simulink model "HW6_Simulink"  (R2019b)
settings: Solver=FixedStepAuto  StartTime=0.0  StopTime=20  RelTol=1e-3
InitFcn:
  | load('BusDefinitions.mat')
undefined symbols (not defined in the file): A1, A1_eval, A2_cont, A2_eval, B1, B1_eval, B2_cont, B2_eval, C1, C1_eval, C2_cont, C2_eval, codertarget, D1, D1_eval, D2_cont, D2_eval, DiscIntNeverNeededParam, Discrete, L1, L2, L3, L4, L5, q1_noise, q2_noise, q3_noise, q4_noise, q5_noise, r1_noise, r2_noise, r3_noise, r4_noise, r5_noise, Time, Ts
libraries: ctrlSharedLib x5, simulink x1
settings Model: ExtModeTrigDuration=80  Creator=Sankalp Bhan  LastModifiedBy=cwhipp
settings DataIOCC: SaveFormat=Structure
settings OptimizationCC: PassReuseOutputArgsThreshold=0  MaxStackSize=64
settings DebuggingCC: ParameterTunabilityLossMsg=error  ArithmeticOperatorsInVariantConditions=warning
settings HardwareCC: ProdBitPerPointer=32  ProdBitPerSizeT=32  ProdBitPerPtrDiffT=32  ProdLargestAtomicInteger=Long  ProdWordSize=32  ProdHWDeviceType=ARM Compatible->ARM 9  UseEmbeddedCoderFeatures=off
settings SFSimCC: SimUseLocalCustomCode=off  MATLABDynamicMemAlloc=off
settings RTWCC: SystemTargetFile=ert.tlc  HardwareBoard=PARROT Mambo  TLCOptions="-aInlineSetEventsForThisBaseRateFcn=TLC_FALSE -aSuppressMultiTaskScheduler=TLC_FALSE   -aRateBasedStepFcn=1"  TemplateMakefile=ert_default_tmf  GenerateReport=on  RTWUseLocalCustomCode=off  Toolchain=Sourcery G++ Lite GNU Toolchain for Drones  LaunchReport=on
settings CodeAppCC: ForceParamTrailComments=on  OperatorAnnotations=on  StateflowObjectComments=on
settings ERTTargetCC: ERTCustomFileBanners=off  MatFileLogging=on  SupportContinuousTime=on  SupportNonInlinedSFcns=on  RemoveResetFunc=off  ModelStepFunctionPrototypeControlCompliant=off

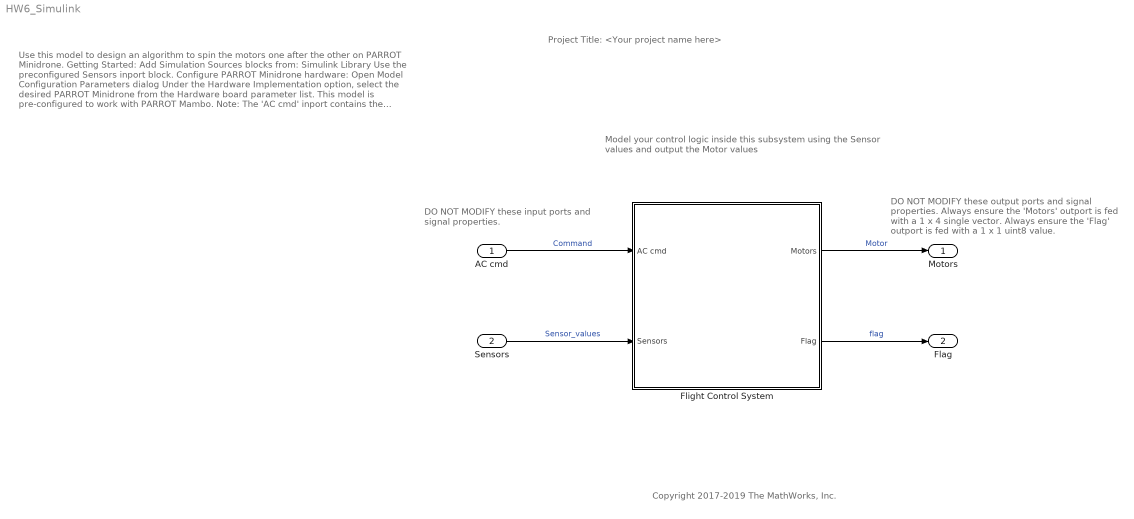
== system HW6_Simulink ==
  note: Model your control logic inside this subsystem
      | using the Sensor values and output the
      | Motor values
  note: DO NOT MODIFY these output ports
      | and signal properties.
      |
      |
      |
      | Always ensure the 'Motors' outport
      | is fed with a 1 x 4 single vector.
      |
      |
      |
      |
      |
      | Always ensure the 'Flag' outport is
      | fed with a 1 x 1 uint8 value.
  note: DO NOT MODIFY these input
      | ports and signal properties.
  note: Copyright 2017-2019 The MathWorks, Inc.
  note: Use this model to design an algorithm to spin the motors one
      | after the other on PARROT Minidrone.
      |
      | Getting Started:
      |
      | Add Simulation Sources blocks from:
      | Simulink Library
      | Use the preconfigured Sensors inport block.
      |
      | Configure PARROT Minidrone hardware:
      |
      | Open Model Configuration Parameters dialog
      |
      | Under the Hardware Implementation option, select the desired
      | PARROT Minidrone from the Hardware board parameter list.
      |
      | This model is pre-configured to work with PARROT Mambo.
      |
      | Note:
      |
      | The 'AC cmd' inport contains the position and orientation
      | reference signals information.
      | The 'Sensors' inport contains data from accelerometer,
      | gyroscope, ultrasonic, pressure and optical flow data.
      | The 'Flag' outport can be used to model an error condition
      | which stops the drone.
      | The 'Motors' outport is fed with the speed values of the 4 motors.
      | Learn more:
      |
      | Simulink Subsystem
      | Simulink Buses
  note: Project Title: <Your project name here>
  AC cmd : Inport  OutDataTypeStr=Bus: CommandBus  BusOutputAsStruct=on
  Sensors : Inport  Port=2  OutDataTypeStr=Bus: SensorsBus  BusOutputAsStruct=on
  Flight Control System : Subsystem  InitFcn=codertarget.parrot.internal.fcsSubsystemCallback(gcb);
  Motors : Outport  OutDataTypeStr=single  PortDimensions=[1 4]  VectorParamsAs1DForOutWhenUnconnected=off
  Flag : Outport  Port=2  OutDataTypeStr=uint8  PortDimensions=1  VectorParamsAs1DForOutWhenUnconnected=off
  wires:
  Flight Control System/1(Motors) -> Motors/1  "Motor"
  AC cmd/1 -> Flight Control System/1(AC cmd)  "Command"
  Sensors/1 -> Flight Control System/2(Sensors)  "Sensor_values"
  Flight Control System/2(Flag) -> Flag/1  "flag"

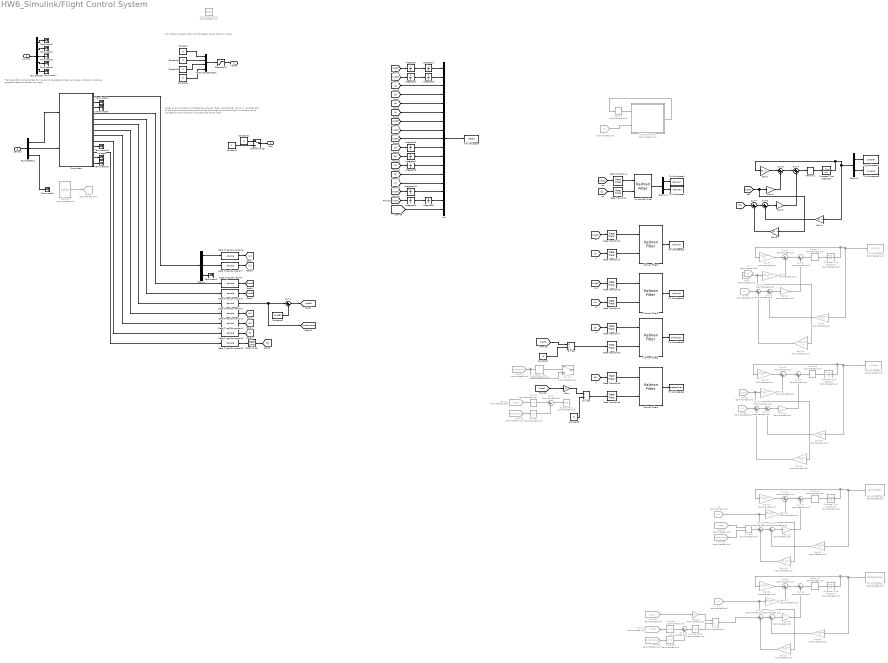
== system HW6_Simulink/Flight Control System ==
  note: The 'Motors' outport is fed with the speed values of the 4 motors.
  note: Model an error condition and feed the value to 'Flag' outport block.
      | Value '0' indicates that all the flight conditions are good and the drone
      | can continue its flight.
      | A non-zero value indicates an error condition, and stops the drone
      | flight.
  note: The SensorsBus contains data from sensors like
      | accelerometer, gyroscope, ultrasonic, pressure,
      | magnetometer and optical flow data.
  AC cmd : Inport
  Sensors : Inport  Port=2
  Bus Selector : BusSelector  OutputSignals=controlModePosVSOrient,pos_ref,takeoff_flag,orient_ref,live_time_ticks
  Bus Selector1 : BusSelector  OutputSignals=VisionSensors,HALSensors,SensorCalibration
  Constant{,3..5} (4 alike) : Constant  Value=0  SampleTime=0.005
  Constant1 : Constant  OutDataTypeStr=uint8
  Constant2 : Constant  Value=0  OutDataTypeStr=uint8
  Constant6 : Constant  Value=-9.4351
  Constant7 : Constant  Value=3
  Constant8 : Constant  Value=3
  Data Type Conversion{,1..8} (9 alike) : DataTypeConversion  OutDataTypeStr=double
  Demux : Demux  Outputs=3
  Demux1 : Demux  Outputs=2
  Demux2 : Demux  Outputs=2
  Discrete-Time Integrator : DiscreteIntegrator  IntegratorMethod=Integration: Backward Euler  SampleTime=-1  ICPrevOutput=DiscIntNeverNeededParam  ICPrevScaledInput=DiscIntNeverNeededParam
  Discrete-Time Integrator{1..4} (4 alike) : DiscreteIntegrator  Commented=on  IntegratorMethod=Integration: Backward Euler  SampleTime=-1  ICPrevOutput=DiscIntNeverNeededParam  ICPrevScaledInput=DiscIntNeverNeededParam
  Divide : Product  Inputs=*/
  Divide1 : Product  Inputs=*/
  Divide2 : Product  Commented=on  Inputs=*/
  Divide4 : Product  Commented=on  Inputs=*/
  From17 : From  Commented=on  GotoTag=vdot
  From{20,22..23,28} (4 alike) : From  Commented=on  GotoTag=wdotnobias
  From21 : From  Commented=on  GotoTag=vdot
  From26 : From  Commented=on  GotoTag=udot
  From27 : From  Commented=on  GotoTag=vdot
  Gain : Gain  Gain=-1
  Gain1 : Gain  Gain=A1  Multiplication=Matrix(K*u)
  Gain{10..11,16,21} (4 alike) : Gain  Commented=on  Gain=D2_cont  Multiplication=Matrix(K*u)
  Gain{5,12,17,22} (4 alike) : Gain  Commented=on  Gain=A2_cont  Multiplication=Matrix(K*u)
  Gain{7,13,18,23} (4 alike) : Gain  Commented=on  Gain=B2_cont  Multiplication=Matrix(K*u)
  Gain14 : Gain  Commented=on  Gain=L3  Multiplication=Matrix(K*u)
  Gain{9,15,20,25} (4 alike) : Gain  Commented=on  Gain=C2_cont  Multiplication=Matrix(K*u)
  Gain19 : Gain  Commented=on  Gain=L4  Multiplication=Matrix(K*u)
  Gain2 : Gain  Gain=B1  Multiplication=Matrix(K*u)
  Gain24 : Gain  Commented=on  Gain=L5  Multiplication=Matrix(K*u)
  Gain26 : Gain  Commented=on  Gain=-1
  Gain3 : Gain  Gain=L1  Multiplication=Matrix(K*u)
  Gain4 : Gain  Gain=C1  Multiplication=Matrix(K*u)
  Gain6 : Gain  Gain=D1  Multiplication=Matrix(K*u)
  Gain8 : Gain  Commented=on  Gain=L2  Multiplication=Matrix(K*u)
  Goto9 : Goto  Commented=on  GotoTag=azbias
  Integrator{,1..8,11} (10 alike) : Integrator
  Interval Test : simulink/Logic and Bit Operations/Interval Test  Commented=on  IntervalClosedRight=on  uplimit=0.5  IntervalClosedLeft=on  lowlimit=-0.5  OutDataTypeStr=boolean
  Kalman Filter1 : ctrlSharedLib/Kalman Filter  TimeDomain=Discrete-Time  UseCurrentEstimator=on  ModelSource=Individual A, B, C, D matrices  ModelSourceVariable=ss(0.95,1,1,0,1)  A=A2_eval  B=B2_eval  C=C2_eval  D=D2_eval  NumberOfStates=1  NumberOfInputs=1  NumberOfOutputs=1  InitialEstimateSource=Dialog  X0=[0]  P0=10  UseK=off  UseGH=off  NumberOfProcessNoiseInputs=1  G=1  TimeInvariantG=on  H=0  TimeInvariantH=on  Q=q2_noise;  TimeInvariantQ=on  R=r2_noise;  TimeInvariantR=on  N=0  TimeInvariantN=on  AddInputPort=on  AddEnablePort=off  OutputEstimatedY=off  OutputP=off  Ts=-1
      settings: SourceProductBaseCode=CT
  Kalman Filter2 : ctrlSharedLib/Kalman Filter  TimeDomain=Discrete-Time  UseCurrentEstimator=on  ModelSource=Individual A, B, C, D matrices  ModelSourceVariable=ss(0.95,1,1,0,1)  A=A2_eval  B=B2_eval  C=C2_eval  D=D2_eval  NumberOfStates=1  NumberOfInputs=1  NumberOfOutputs=1  InitialEstimateSource=Dialog  X0=[0]  P0=10  UseK=off  UseGH=off  NumberOfProcessNoiseInputs=1  G=1  TimeInvariantG=on  H=0  TimeInvariantH=on  Q=q3_noise;  TimeInvariantQ=on  R=r3_noise;  TimeInvariantR=on  N=0  TimeInvariantN=on  AddInputPort=on  AddEnablePort=off  OutputEstimatedY=off  OutputP=off  Ts=-1
      settings: SourceProductBaseCode=CT
  Kalman Filter3 : ctrlSharedLib/Kalman Filter  TimeDomain=Discrete-Time  UseCurrentEstimator=on  ModelSource=Individual A, B, C, D matrices  ModelSourceVariable=ss(0.95,1,1,0,1)  A=A2_eval  B=B2_eval  C=C2_eval  D=D2_eval  NumberOfStates=1  NumberOfInputs=1  NumberOfOutputs=1  InitialEstimateSource=Dialog  X0=[0]  P0=10  UseK=off  UseGH=off  NumberOfProcessNoiseInputs=1  G=1  TimeInvariantG=on  H=0  TimeInvariantH=on  Q=q4_noise;  TimeInvariantQ=on  R=r4_noise;  TimeInvariantR=on  N=0  TimeInvariantN=on  AddInputPort=on  AddEnablePort=off  OutputEstimatedY=off  OutputP=off  Ts=-1
      settings: SourceProductBaseCode=CT
  Kalman Filter4 : ctrlSharedLib/Kalman Filter  TimeDomain=Discrete-Time  UseCurrentEstimator=on  ModelSource=Individual A, B, C, D matrices  ModelSourceVariable=ss(0.95,1,1,0,1)  A=A2_eval  B=B2_eval  C=C2_eval  D=D2_eval  NumberOfStates=1  NumberOfInputs=1  NumberOfOutputs=1  InitialEstimateSource=Dialog  X0=[0]  P0=10  UseK=off  UseGH=off  NumberOfProcessNoiseInputs=1  G=1  TimeInvariantG=on  H=0  TimeInvariantH=on  Q=q5_noise;  TimeInvariantQ=on  R=r5_noise;  TimeInvariantR=on  N=0  TimeInvariantN=on  AddInputPort=on  AddEnablePort=off  OutputEstimatedY=off  OutputP=off  Ts=-1
      settings: SourceProductBaseCode=CT
  MATLAB Function : MATLAB Function  Commented=on  TreatAsAtomicUnit=on
  Manual Switch : ManualSwitch
  Memory{,2..5} (5 alike) : Memory  Commented=on
  Memory1 : Memory
  Mux : Mux  Inputs=17
  Pulse Generator2 : DiscretePulseGenerator  Commented=on  Amplitude=400  Period=1600  PulseWidth=400  PhaseDelay=1200  SampleTime=Ts
  Rate Limiter : RateLimiter  RisingSlewLimit=50  FallingSlewLimit=-50  SampleTimeMode=inherited
  Rate Transition{,1..9} (10 alike) : RateTransition  OutPortSampleTime=0.005
  Saturation1 : Saturate  UpperLimit=500  LowerLimit=0  OutDataTypeStr=single
  Selector : Selector  Commented=on  InputPortWidth=8  IndexOptions=Index vector (dialog)  Indices=[3]  OutputSizes=1
  Square{,1..3} (4 alike) : Math  Commented=on  Operator=square  SignedPower=off  SaturateOnIntegerOverflow=on
  Square Root : Sqrt  Commented=on  SaturateOnIntegerOverflow=on
  Square Root1 : Sqrt  Commented=on  SaturateOnIntegerOverflow=on
  Subsystem : Subsystem
  Sum1 : Sum  Inputs=|+-
  Sum{9..11,14..15,18..19,22} (8 alike) : Sum  Commented=on  Inputs=|+-
  Sum{2,6,8,12..13,16..17,20..21,23} (10 alike) : Sum  Commented=on  Inputs=|++
  Sum3 : Sum  Inputs=|++
  Sum4 : Sum  Inputs=|++
  Sum5 : Sum  Inputs=|+-
  Sum7 : Sum  Inputs=|+-
  Switch : Switch  Commented=on  Criteria=u2 > Threshold
  Terminator{1..9,15,18} (11 alike) : Terminator
  To Workspace : ToWorkspace  VariableName=states  SaveFormat=Structure With Time  SampleTime=-1
  To Workspace1 : ToWorkspace  VariableName=zkalman  SaveFormat=Structure With Time  SampleTime=-1
  To Workspace10 : ToWorkspace  Commented=on  VariableName=vwiener  SaveFormat=Structure With Time  SampleTime=-1
  To Workspace11 : ToWorkspace  Commented=on  VariableName=phiwiener  SaveFormat=Structure With Time  SampleTime=-1
  To Workspace12 : ToWorkspace  Commented=on  VariableName=thetawiener  SaveFormat=Structure With Time  SampleTime=-1
  To Workspace2 : ToWorkspace  VariableName=wkalman  SaveFormat=Structure With Time  SampleTime=-1
  To Workspace3 : ToWorkspace  VariableName=ukalman  SaveFormat=Structure With Time  SampleTime=-1
  To Workspace4 : ToWorkspace  VariableName=vkalman  SaveFormat=Structure With Time  SampleTime=-1
  To Workspace5 : ToWorkspace  VariableName=phikalman  SaveFormat=Structure With Time  SampleTime=-1
  To Workspace6 : ToWorkspace  VariableName=thetakalman  SaveFormat=Structure With Time  SampleTime=-1
  To Workspace7 : ToWorkspace  VariableName=zwiener  SaveFormat=Structure With Time  SampleTime=-1
  To Workspace8 : ToWorkspace  VariableName=wwiener  SaveFormat=Structure With Time  SampleTime=-1
  To Workspace9 : ToWorkspace  Commented=on  VariableName=uwiener  SaveFormat=Structure With Time  SampleTime=-1
  Vector Concatenate1 : Concatenate  NumInputs=4
  hello : From  Commented=on  GotoTag=udot
  hello1 : From  Commented=on  GotoTag=vdot
  its me : From  Commented=on  GotoTag=u
  its me1 : From  Commented=on  GotoTag=v
  p1 : From  Commented=on  GotoTag=p
  p2 : From  Commented=on  GotoTag=p
  q1 : From  Commented=on  GotoTag=q
  voltage : Terminator
  z : From  Commented=on  GotoTag=h
  zw Kalman Filter : ctrlSharedLib/Kalman Filter  TimeDomain=Discrete-Time  UseCurrentEstimator=on  ModelSource=Individual A, B, C, D matrices  ModelSourceVariable=ss(0.95,1,1,0,1)  A=A1_eval  B=B1_eval  C=C1_eval  D=D1_eval  NumberOfStates=1  NumberOfInputs=1  NumberOfOutputs=1  InitialEstimateSource=Dialog  X0=[0;0 ]  P0=10  UseK=off  UseGH=off  NumberOfProcessNoiseInputs=1  G=1  TimeInvariantG=on  H=0  TimeInvariantH=on  Q=[0 0 ; 0 1].*q1_noise;  TimeInvariantQ=on  R=r1_noise;  TimeInvariantR=on  N=0  TimeInvariantN=on  AddInputPort=on  AddEnablePort=off  OutputEstimatedY=off  OutputP=off  Ts=-1
      settings: SourceProductBaseCode=CT
  Motors : Outport  VectorParamsAs1DForOutWhenUnconnected=off
  Flag : Outport  Port=2  VectorParamsAs1DForOutWhenUnconnected=off
  wires:
  AC cmd/1 -> Bus Selector/1
  Sensors/1 -> Bus Selector1/1
  Bus Selector/1 -> Terminator3/1  "<controlModePosVSOrient>"
  Bus Selector/2 -> Terminator4/1  "<pos_ref>"
  Bus Selector/3 -> Terminator5/1  "<takeoff_flag>"
  Bus Selector/4 -> Terminator6/1  "<orient_ref>"
  Bus Selector/5 -> Terminator7/1  "<live_time_ticks>"
  Manual Switch/1 -> Flag/1
  Constant2/1 -> Manual Switch/1
  Constant1/1 -> Manual Switch/2
  Vector Concatenate1/1 -> Saturation1/1
  Constant/1 -> Vector Concatenate1/1
  Constant4/1 -> Vector Concatenate1/4
  Constant5/1 -> Vector Concatenate1/2
  Constant3/1 -> Vector Concatenate1/3
  Saturation1/1 -> Motors/1
  Bus Selector1/1 -> Subsystem/1(<VisionSensors>)  "<VisionSensors>"
  Bus Selector1/2 -> Subsystem/2(<HALSensors>)  "<HALSensors>"
  Subsystem/1(OF_data) -> Demux/1
  Subsystem/2(posVIS_data) -> Terminator2/1
  Subsystem/3(usePosVIS_flag) -> Terminator8/1
  Subsystem/10(prs) -> Terminator15/1
  Subsystem/11(altitude_sonar) -> Data Type Conversion8/1
  Subsystem/13(vbat_percentage) -> Terminator18/1
  [udot] -> Integrator/1
  Integrator/1 -> Integrator1/1
  Integrator2/1 -> Integrator3/1
  [vdot] -> Integrator2/1
  [r] -> Integrator8/1
  [p] -> Integrator6/1
  [q] -> Integrator7/1
  [wdot] -> Integrator11/1
  [z] -> Mux/3  "Zned"
  Integrator3/1 -> Mux/2  "Yned"
  Integrator1/1 -> Mux/1  "Xned"
  [p] -> Mux/4
  [q] -> Mux/5
  Subsystem/4(ddx) -> Data Type Conversion/1
  Data Type Conversion/1 -> [udot]
  Subsystem/5(ddy) -> Data Type Conversion1/1
  Data Type Conversion1/1 -> [vdot]
  Subsystem/6(ddz) -> Data Type Conversion2/1
  Data Type Conversion2/1 -> Sum1/1, [wdotnobias]
  Subsystem/7(p) -> Data Type Conversion3/1
  Data Type Conversion3/1 -> [p]
  Subsystem/8(q) -> Data Type Conversion4/1
  Data Type Conversion4/1 -> [q]
  Subsystem/9(r) -> Data Type Conversion5/1
  Data Type Conversion5/1 -> [r]
  Data Type Conversion7/1 -> [v]
  Data Type Conversion6/1 -> [u]
  Demux/1 -> Data Type Conversion6/1
  Demux/2 -> Data Type Conversion7/1
  Demux/3 -> Terminator1/1
  Subsystem/12(vbat_V) -> voltage/1
  Mux/1 -> To Workspace/1
  Integrator6/1 -> Mux/10  "phi"
  Integrator7/1 -> Mux/11  "theta"
  Integrator8/1 -> Mux/12  "psi"
  Integrator11/1 -> Mux/15
  [udot] -> Mux/7
  [vdot] -> Mux/8
  [r] -> Mux/6
  [u] -> Mux/13
  [v] -> Mux/14
  Demux1/2 -> To Workspace2/1  "w"
  Rate Transition1/1 -> zw Kalman Filter/1
  Rate Transition/1 -> zw Kalman Filter/2
  zw Kalman Filter/1 -> Demux1/1
  Demux1/1 -> To Workspace1/1  "z"
  [wdot] -> Rate Transition1/1
  MATLAB Function/1(z_currentmod) -> Memory/1
  [udot] -> Rate Transition3/1
  [u] -> Rate Transition2/1
  Rate Transition3/1 -> Kalman Filter1/1
  Rate Transition2/1 -> Kalman Filter1/2
  Kalman Filter1/1 -> To Workspace3/1  "z"
  Integrator4/1 -> Integrator5/1
  [wdot] -> Integrator4/1
  Integrator5/1 -> Mux/16  "Yned"
  Selector/1 -> Goto9/1
  [wdot] -> Mux/9
  Constant6/1 -> Sum1/2
  Sum1/1 -> [wdot]
  z/1 -> MATLAB Function/2(z_current)
  Memory/1 -> MATLAB Function/1(z_last)
  [vdot] -> Divide/1
  Divide/1 -> Rate Transition6/1  "phi"
  From21/1 -> Square/1
  From22/1 -> Square1/1
  Square/1 -> Sum2/1
  Square1/1 -> Sum2/2
  Sum2/1 -> Square Root/1
  [udot] -> Gain/1
  Gain/1 -> Divide1/1
  Divide1/1 -> Rate Transition8/1  "theta"
  [vdot] -> Rate Transition5/1
  Rate Transition4/1 -> Kalman Filter2/2
  [v] -> Rate Transition4/1
  Kalman Filter2/1 -> To Workspace4/1  "z"
  Rate Transition5/1 -> Kalman Filter2/1
  Kalman Filter3/1 -> To Workspace5/1  "z"
  Rate Transition7/1 -> Kalman Filter3/1
  [p] -> Rate Transition7/1
  Rate Transition6/1 -> Kalman Filter3/2
  Rate Transition8/1 -> Kalman Filter4/2
  Rate Transition9/1 -> Kalman Filter4/1
  [q] -> Rate Transition9/1
  Kalman Filter4/1 -> To Workspace6/1  "z"
  Gain1/1 -> Sum3/1  "Axe"
  Sum3/1 -> Sum4/1
  Discrete-Time Integrator/1 -> Gain1/1, Gain4/1, Demux2/1  "xe"
  Gain2/1 -> Sum3/2  "Bu"
  [wdot] -> Gain6/1, Gain2/1  "u"
  Sum5/1 -> Gain3/1
  Gain3/1 -> Sum4/2  "L(y-Cx-Du)"
  Gain4/1 -> Sum5/2  "Cx"
  [h] -> Sum7/1
  Sum7/1 -> Sum5/1
  Gain6/1 -> Sum7/2  "Du"
  Sum4/1 -> Memory1/1
  Memory1/1 -> Discrete-Time Integrator/1
  Demux2/1 -> To Workspace7/1
  Demux2/2 -> To Workspace8/1
  Gain7/1 -> Sum6/2  "Bu"
  Gain9/1 -> Sum9/2  "Cx"
  its me/1 -> Sum10/1
  Gain10/1 -> Sum10/2  "Du"
  Sum10/1 -> Sum9/1
  Sum9/1 -> Gain8/1
  hello/1 -> Gain10/1, Gain7/1  "u"
  Gain5/1 -> Sum6/1  "Axe"
  Sum6/1 -> Sum8/1
  Gain8/1 -> Sum8/2  "L(y-Cx-Du)"
  Sum8/1 -> Memory2/1
  Memory2/1 -> Discrete-Time Integrator1/1
  Discrete-Time Integrator1/1 -> Gain5/1, Gain9/1, To Workspace9/1  "xe"
  hello1/1 -> Gain11/1, Gain13/1  "u"
  Gain11/1 -> Sum11/2  "Du"
  Sum11/1 -> Sum14/1
  its me1/1 -> Sum11/1
  Gain15/1 -> Sum14/2  "Cx"
  Gain13/1 -> Sum12/2  "Bu"
  Discrete-Time Integrator2/1 -> Gain12/1, Gain15/1, To Workspace10/1  "xe"
  Sum12/1 -> Sum13/1
  Sum13/1 -> Memory3/1
  Gain12/1 -> Sum12/1  "Axe"
  Sum14/1 -> Gain14/1
  Memory3/1 -> Discrete-Time Integrator2/1
  Gain14/1 -> Sum13/2  "L(y-Cx-Du)"
  Sum18/1 -> Gain19/1
  Gain19/1 -> Sum17/2  "L(y-Cx-Du)"
  Memory4/1 -> Discrete-Time Integrator3/1
  Discrete-Time Integrator3/1 -> Gain17/1, To Workspace11/1, Gain20/1  "xe"
  Gain17/1 -> Sum16/1  "Axe"
  Gain18/1 -> Sum16/2  "Bu"
  Gain20/1 -> Sum18/2  "Cx"
  Gain16/1 -> Sum15/2  "Du"
  Sum16/1 -> Sum17/1
  Sum17/1 -> Memory4/1
  Divide2/1 -> Sum15/1
  p2/1 -> Gain16/1, Gain18/1  "u"
  Sum15/1 -> Sum18/1
  From23/1 -> Divide2/2
  From17/1 -> Divide2/1
  Sum19/1 -> Sum22/1
  Gain23/1 -> Sum20/2  "Bu"
  Discrete-Time Integrator4/1 -> Gain22/1, To Workspace12/1, Gain25/1  "xe"
  Gain21/1 -> Sum19/2  "Du"
  Gain25/1 -> Sum22/2  "Cx"
  Gain22/1 -> Sum20/1  "Axe"
  Sum21/1 -> Memory5/1
  Sum20/1 -> Sum21/1
  Sum22/1 -> Gain24/1
  Gain24/1 -> Sum21/2  "L(y-Cx-Du)"
  q1/1 -> Gain21/1, Gain23/1  "u"
  Memory5/1 -> Discrete-Time Integrator4/1
  From27/1 -> Square2/1
  Sum23/1 -> Square Root1/1
  Square3/1 -> Sum23/2
  Divide4/1 -> Sum19/1  "theta"
  From26/1 -> Gain26/1
  From28/1 -> Square3/1
  Gain26/1 -> Divide4/1
  Square2/1 -> Sum23/1
  Square Root1/1 -> Divide4/2
  [wdotnobias] -> Mux/17
  [z] -> Rate Transition/1
  Bus Selector1/3 -> Terminator9/1  "<SensorCalibration>"
  Data Type Conversion8/1 -> Rate Limiter/1
  Rate Limiter/1 -> [z]
  Constant7/1 -> Divide/2
  Constant8/1 -> Divide1/2
  Interval Test/1 -> Switch/2
  From20/1 -> Switch/3, Interval Test/1

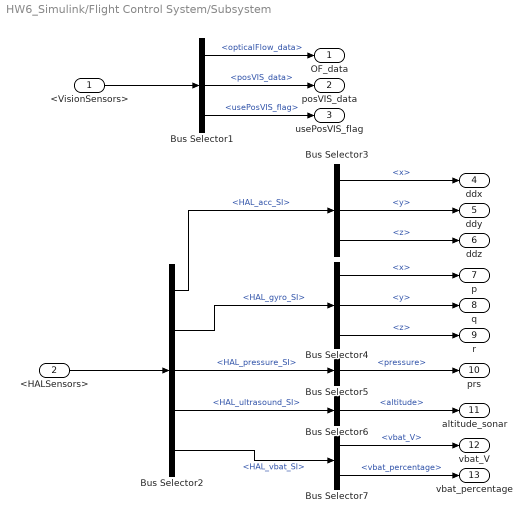
== system HW6_Simulink/Flight Control System/Subsystem ==
  <VisionSensors> : Inport
  <HALSensors> : Inport  Port=2
  Bus Selector1 : BusSelector  OutputSignals=opticalFlow_data,posVIS_data,usePosVIS_flag
  Bus Selector2 : BusSelector  OutputSignals=HAL_acc_SI,HAL_gyro_SI,HAL_pressure_SI,HAL_ultrasound_SI,HAL_vbat_SI
  Bus Selector3 : BusSelector  OutputSignals=x,y,z
  Bus Selector4 : BusSelector  OutputSignals=x,y,z
  Bus Selector5 : BusSelector  OutputSignals=pressure
  Bus Selector6 : BusSelector  OutputSignals=altitude
  Bus Selector7 : BusSelector  OutputSignals=vbat_V,vbat_percentage
  OF_data : Outport  VectorParamsAs1DForOutWhenUnconnected=off
  posVIS_data : Outport  Port=2  VectorParamsAs1DForOutWhenUnconnected=off
  usePosVIS_flag : Outport  Port=3  VectorParamsAs1DForOutWhenUnconnected=off
  ddx : Outport  Port=4  VectorParamsAs1DForOutWhenUnconnected=off
  ddy : Outport  Port=5  VectorParamsAs1DForOutWhenUnconnected=off
  ddz : Outport  Port=6  VectorParamsAs1DForOutWhenUnconnected=off
  p : Outport  Port=7  VectorParamsAs1DForOutWhenUnconnected=off
  q : Outport  Port=8  VectorParamsAs1DForOutWhenUnconnected=off
  r : Outport  Port=9  VectorParamsAs1DForOutWhenUnconnected=off
  prs : Outport  Port=10  VectorParamsAs1DForOutWhenUnconnected=off
  altitude_sonar : Outport  Port=11  VectorParamsAs1DForOutWhenUnconnected=off
  vbat_V : Outport  Port=12  VectorParamsAs1DForOutWhenUnconnected=off
  vbat_percentage : Outport  Port=13  VectorParamsAs1DForOutWhenUnconnected=off
  wires:
  <VisionSensors>/1 -> Bus Selector1/1
  <HALSensors>/1 -> Bus Selector2/1
  Bus Selector1/1 -> OF_data/1  "<opticalFlow_data>"
  Bus Selector1/2 -> posVIS_data/1  "<posVIS_data>"
  Bus Selector1/3 -> usePosVIS_flag/1  "<usePosVIS_flag>"
  Bus Selector2/1 -> Bus Selector3/1  "<HAL_acc_SI>"
  Bus Selector2/2 -> Bus Selector4/1  "<HAL_gyro_SI>"
  Bus Selector2/3 -> Bus Selector5/1  "<HAL_pressure_SI>"
  Bus Selector2/4 -> Bus Selector6/1  "<HAL_ultrasound_SI>"
  Bus Selector2/5 -> Bus Selector7/1  "<HAL_vbat_SI>"
  Bus Selector3/1 -> ddx/1  "<x>"
  Bus Selector3/2 -> ddy/1  "<y>"
  Bus Selector3/3 -> ddz/1  "<z>"
  Bus Selector4/2 -> q/1  "<y>"
  Bus Selector4/1 -> p/1  "<x>"
  Bus Selector4/3 -> r/1  "<z>"
  Bus Selector5/1 -> prs/1  "<pressure>"
  Bus Selector6/1 -> altitude_sonar/1  "<altitude>"
  Bus Selector7/1 -> vbat_V/1  "<vbat_V>"
  Bus Selector7/2 -> vbat_percentage/1  "<vbat_percentage>"

== matlab function HW6_Simulink/Flight Control System/MATLAB Function ==
  data: z_last input; z_currentmod output; z_current input
function z_currentmod  = fcn(z_last, z_current)

if z_current > 0.43
    if abs(z_current - z_last) > 0.1
        z_currentmod = z_last;
    else
        z_currentmod = z_current;
    end
        

else 
    z_currentmod = z_current;
end
